simulink model "sldemo_pid2dof"  (R2017a)
settings: Solver=ode45  StartTime=0.0  StopTime=50  RelTol=1e-5  EnableMultiTasking=on
undefined symbols (not defined in the file): sigbuilder_block
libraries: simulink x1
settings Model: Creator=The MathWorks, Inc.  LastModifiedBy=rj2318
settings DataIOCC: LimitDataPoints=on  SaveFormat=Array
settings OptimizationCC: ExpressionDepthLimit=2147483647  LifeSpan=inf
settings DebuggingCC: UnderspecifiedInitializationDetection=Classic  MergeDetectMultiDrivingBlocksExec=none  FcnCallInpInsideContextMsg=warning  AllowSymbolicDim=off  StateNameClashWarn=warning  SFUnexpectedBacktrackingDiag=warning  SFNoUnconditionalDefaultTransitionDiag=warning  SFExecutionAtInitializationDiag=none
settings HardwareCC: ProdBitPerPointer=32  ProdBitPerSizeT=32  ProdBitPerPtrDiffT=32  ProdLargestAtomicFloat=None  ProdIntDivRoundTo=Undefined  ProdEndianess=Unspecified  ProdWordSize=32  ProdHWDeviceType=32-bit Generic
settings ModelReferenceCC: PropagateSignalLabelsOutOfModel=off
settings GRTTargetCC: TargetLangStandard=C89/C90 (ANSI)  GeneratePreprocessorConditionals=Disable all  CombineOutputUpdateFcns=off  GRTInterface=on
settings ConfigComp: CovMetricSettings=dw  CovHtmlReporting=on  CovSaveCumulativeToWorkspaceVar=on  CovSaveSingleToWorkspaceVar=on  CovExternalEMLEnable=off  CovSFcnEnable=off

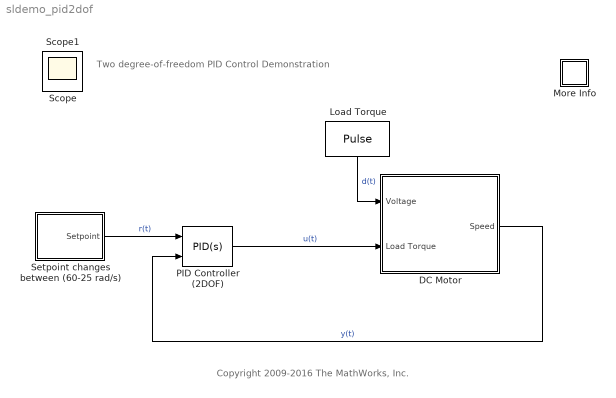
== system sldemo_pid2dof ==
  note: Two degree-of-freedom PID Control Demonstration
  note: Copyright 2009-2016 The MathWorks, Inc.
  DC Motor : Subsystem  mask(DC Motor){R=2, L=0.5, Km=0.1, Kf=0.2, J=0.02, Kb=0.1}
      mask prompts: R "R (Ohms)"; L "L (Henrys)"; Km "Km (Torque Constant)"; Kf "Kf (Nms)"; J "J (kg.m^2/s^2)"; Kb "Kb (Back emf Constant)"
      mask help: An ideal model of a DC Motor
      mask Help: This is <b>more elaborate<b> help.
      mask Display: image(fullfile(matlabroot,'toolbox','simulink','simdemos','industrial','images','maskIconDCMotor.png'))
  Load Torque : DiscretePulseGenerator  PulseType=Time based  Amplitude=-5  Period=10  PulseWidth=50  PhaseDelay=5
  More Info : Subsystem
      settings: OpenFcn=showdemo('sldemo_pid2dof')
      mask Display: disp('?')
  PID Controller (2DOF) : simulink/Continuous/PID Controller (2DOF)  Tag=PID1  Controller=PID  TimeDomain=Continuous-time  SampleTime=-1  IntegratorMethod=Forward Euler  FilterMethod=Forward Euler  Form=Parallel  UseFilter=on  ControllerParametersSource=internal  P=0.2  I=1.0  D=0.06  N=12  b=1  c=1  InitialConditionSource=internal  InitialConditionForIntegrator=0  InitialConditionForFilter=0  ExternalReset=none  ZeroCross=off  LimitOutput=off  UpperSaturationLimit=inf  LowerSaturationLimit=-inf  LinearizeAsGain=off  AntiWindupMode=none  Kb=1  TrackingMode=off  Kt=1  PParamMin=[]  PParamMax=[]  IParamMin=[]  IParamMax=[]  DParamMin=[]  DParamMax=[]  NParamMin=[]  NParamMax=[]  bParamMin=[]  bParamMax=[]  cParamMin=[]  cParamMax=[]  KbParamMin=[]  KbParamMax=[]  KtParamMin=[]  KtParamMax=[]  POutMin=[]  POutMax=[]  IOutMin=[]  IOutMax=[]  DOutMin=[]  DOutMax=[]  NOutMin=[]  NOutMax=[]  bOutMin=[]  bOutMax=[]  cOutMin=[]  cOutMax=[]  KbOutMin=[]  KbOutMax=[]  KtOutMin=[]  KtOutMax=[]  IntegratorOutMin=[]  IntegratorOutMax=[]  FilterOutMin=[]  FilterOutMax=[]  SumOutMin=[]  SumOutMax=[]  Sum1OutMin=[]  Sum1OutMax=[]  Sum2OutMin=[]  Sum2OutMax=[]  Sum3OutMin=[]  Sum3OutMax=[]  SumI1OutMin=[]  SumI1OutMax=[]  SumI2OutMin=[]  SumI2OutMax=[]  SumI3OutMin=[]  SumI3OutMax=[]  SumDOutMin=[]  SumDOutMax=[]  SaturationOutMin=[]  SaturationOutMax=[]  IntegratorContinuousStateAttributes=''  IntegratorStateMustResolveToSignalObject=off  IntegratorRTWStateStorageClass=Auto  FilterContinuousStateAttributes=''  FilterStateMustResolveToSignalObject=off  FilterRTWStateStorageClass=Auto  DifferentiatorICPrevScaledInput=0  DifferentiatorOutMin=[]  DifferentiatorOutMax=[]  InitialConditionSetting=State (most efficient)
  Setpoint changes between (60-25 rad/s) : Subsystem  Tag=STV Subsys  LoadFcn=sigbuilder_block('load');  StartFcn=sigbuilder_block('start');  StopFcn=sigbuilder_block('stop');  ClipboardFcn=sigbuilder_block('clipboard');  mask(Sigbuilder block){tuvar=[0:10]}
      mask help: Create and generate interchangeable groups of signals whose waveforms are piecewise linear.
      mask init:
      | if ~strcmp(get_param(bdroot(gcbh),'SimulationStatus'),'stopped') tuvar = sigbuilder_block('maskInit'); end
      settings: CopyFcn=sigbuilder_block('copy');  DeleteFcn=sigbuilder_block('delete');  ModelCloseFcn=sigbuilder_block('modelClose');  PreSaveFcn=sigbuilder_block('preSave');  PauseFcn=sigbuilder_block('pause')  ContinueFcn=sigbuilder_block('continue')  NameChangeFcn=sigbuilder_block('namechange');  OpenFcn=sigbuilder_block('open',[312.75 282 550.5 399.75 ]);  CloseFcn=sigbuilder_block('close');
      mask Display: plot(0, 0, 100, 100,[2, 2, 32, 32, 2], [68, 8, 8, 68, 68],[32, 2], [38, 38], [32, 19, 2],[53, 60, 44], [32, 17, 17, 2],[16, 16, 31, 31]);txt = getActiveGroup(gcbh);text(2, 100, txt,'verticalAlignment', 'top');
  Scope : Scope
  Scope1 : Scope
  wires:
  PID Controller (2DOF)/1 -> DC Motor/2(Load Torque)  "u(t)"
  Load Torque/1 -> DC Motor/1(Voltage)  "d(t)"
  Setpoint changes between (60-25 rad/s)/1(Setpoint) -> PID Controller (2DOF)/1  "r(t)"
  DC Motor/1(Speed) -> PID Controller (2DOF)/2  "y(t)"

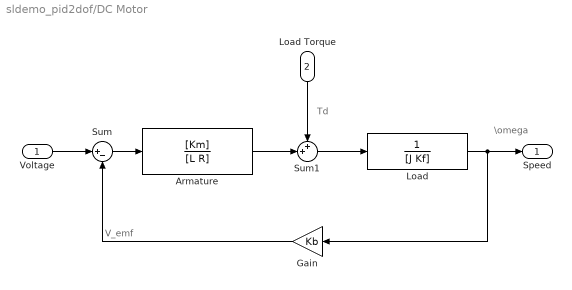
== system sldemo_pid2dof/DC Motor ==
  note: \omega
  note: V_emf
  note: Td
  Voltage : Inport
  Load Torque : Inport  Port=2
  Armature : TransferFcn  Numerator=[Km]  Denominator=[L R]
  Gain : Gain  Gain=Kb
  Load : TransferFcn  Denominator=[J Kf]
  Sum : Sum  Inputs=|+-
  Sum1 : Sum  Inputs=++|
  Speed : Outport
  wires:
  Load/1 -> Speed/1, Gain/1
  Load Torque/1 -> Sum1/1
  Armature/1 -> Sum1/2
  Sum1/1 -> Load/1
  Sum/1 -> Armature/1
  Voltage/1 -> Sum/1
  Gain/1 -> Sum/2

== system sldemo_pid2dof/More Info ==

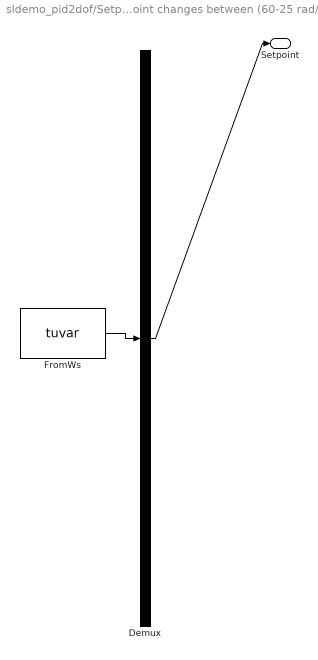
== system sldemo_pid2dof/Setpoint changes between (60-25 rad//s) ==
  Demux : Demux  Tag=STV Demux  Outputs=1
  FromWs : FromWorkspace  Tag=STV FromWs  VariableName=tuvar  SampleTime=0
      SigBuilderData=|
      | common.afterFinalStr = 'Extrapolate'
      | common.sampleTime = 0
      | dataSet.timeRange = [0 50]
      | dataSet.name = 'Group 1'
      | sbobj.Groups.Name = 'Group 1'
      | sbobj.Groups.Signals.Name = 'Setpoint'
      | sbobj.Groups.Signals.XData = [0 10 10 20 20 29.9 29.9 50]
      | sbobj.Groups.Signals.YData = [60 60 25 25 40 40 30 30]
  Setpoint : Outport  Tag=STV Outport
  wires:
  FromWs/1 -> Demux/1
  Demux/1 -> Setpoint/1
